simulink library "Lib_EMTAT"  (R2021b)
settings: Solver=VariableStepAuto  StartTime=0.0  StopTime=10.0  RelTol=1e-3
undefined symbols (not defined in the file or in its folder): A_M, B_M, Cj, component_degradation_input, Cs, E0_M, f_sw, K_M, MWS, Q_M, Q_rr, r_c, r_D, R_M, Rj, Ru, SNR_DX_M, SNR_IC_M, SNR_Mn_M, SNR_Mx_M, SOC_Init_M, u_ce0, u_D0
libraries: $bdroot x82, simulink x23, Lib_Dyn_StateSpace_EMTAT x3, PB_Library_Master_Working x1
(part 4 of 7)

== system Lib_EMTAT/Components/Physics-Based/Electrothermal_Battery_Model ==
  note: Electrical Model
  it_base : Inport
  I_Demand : Inport  Port=2
  Temp (Ra) : Inport  Port=3  Unit=degC
  FaultToggle : Inport  Port=4  Unit=degC
  Battery Core (w/ Q) : Subsystem
  Bus Creator : BusCreator  Inputs=7
  Catastrophic Fault Block{,1..5} (6 alike) : $bdroot/Components/Physics-Based/Catastrophic Fault Block  SystemSampleTime=-1  VariantActivationTime=update diagram  Latency=0  AutoFrameSizeCalculation=off
  Degradation Parameter Multiplier : $bdroot/Components/Physics-Based/Degradation Parameter Multiplier  SystemSampleTime=-1  VariantActivationTime=update diagram  Latency=0  AutoFrameSizeCalculation=off
  Product1 : Product
  Rankine to Celsius : $bdroot/Components/Physics-Based/Rankine to Celsius  SystemSampleTime=-1  VariantActivationTime=update diagram  Latency=0  AutoFrameSizeCalculation=off
  it_Dot = f(i) : Subsystem
  Vout : Outport  VectorParamsAs1DForOutWhenUnconnected=off
  Outputs : Outport  Port=2  VectorParamsAs1DForOutWhenUnconnected=off
  it_Dot : Outport  Port=3  VectorParamsAs1DForOutWhenUnconnected=off
  Heat : Outport  Port=4  VectorParamsAs1DForOutWhenUnconnected=off
  SOC : Outport  Port=5  VectorParamsAs1DForOutWhenUnconnected=off
  it : Outport  Port=6  VectorParamsAs1DForOutWhenUnconnected=off
  wires:
  Rankine to Celsius/1 -> Battery Core (w/ Q)/3(Tavg)
  Battery Core (w/ Q)/3(it) -> Catastrophic Fault Block5/2, Bus Creator/6  "it"
  Battery Core (w/ Q)/2(SOC) -> Catastrophic Fault Block4/2, Bus Creator/4  "SOC"
  it_base/1 -> Battery Core (w/ Q)/1(it_base)
  Battery Core (w/ Q)/1(Vout) -> Catastrophic Fault Block/2, Bus Creator/1, Product1/1  "Vout"
  Product1/1 -> Bus Creator/3  "Pout"
  it_Dot = f(i)/1(it_Dot) -> Catastrophic Fault Block2/2, Bus Creator/5  "it_Dot"
  I_Demand/1 -> it_Dot = f(i)/1(i), Battery Core (w/ Q)/2(I_Demand), Bus Creator/2, Product1/2  "Iout"
  Battery Core (w/ Q)/4(Heat_Generated) -> Catastrophic Fault Block3/2, Bus Creator/7  "Heat_Generated"
  Temp (Ra)/1 -> Rankine to Celsius/1
  Catastrophic Fault Block/1 -> Vout/1
  FaultToggle/1 -> [FT]
  [FT] -> Catastrophic Fault Block/1
  [FT] -> Catastrophic Fault Block1/1
  Bus Creator/1 -> Catastrophic Fault Block1/2
  Catastrophic Fault Block1/1 -> Outputs/1
  [FT] -> Catastrophic Fault Block2/1
  Catastrophic Fault Block2/1 -> it_Dot/1
  [FT] -> Catastrophic Fault Block3/1
  Catastrophic Fault Block3/1 -> Heat/1
  Catastrophic Fault Block4/1 -> SOC/1
  [FT] -> Catastrophic Fault Block4/1
  Catastrophic Fault Block5/1 -> it/1
  [FT] -> Catastrophic Fault Block5/1

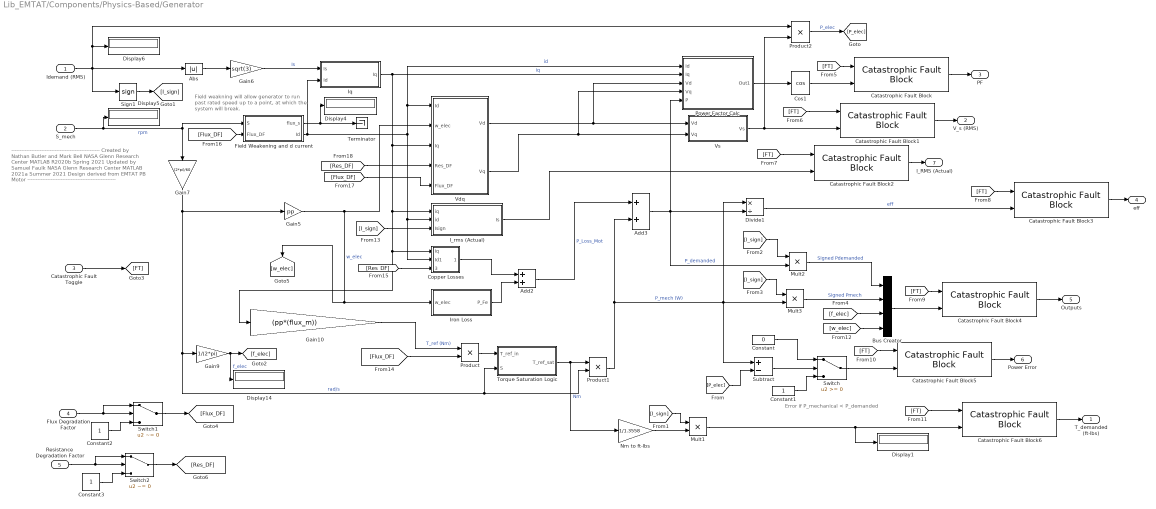
== system Lib_EMTAT/Components/Physics-Based/Generator ==
  note: Field weakning will allow generator to run past rated speed up to a point, at which the system will break.
  note: Error if P_mechanical < P_demanded
  note: -----------------------------------------------------
      | Created by Nathan Butler and Mark Bell
      | NASA Glenn Research Center
      | MATLAB R2020b
      | Spring 2021
      |
      | Updated by Samuel Faulk
      | NASA Glenn Research Center
      | MATLAB 2021a
      | Summer 2021
      |
      | Design derived from EMTAT PB Motor
      | -----------------------------------------------------
  Idemand (RMS) : Inport
  S_mech : Inport  Port=2
  Catastrophic Fault Toggle : Inport  Port=3
  Flux Degradation Factor : Inport  Port=4
  Resistance Degradation Factor : Inport  Port=5
  Abs : Abs
  Add2 : Sum
  Add3 : Sum
  Bus Creator : BusCreator  Inputs=4
  Catastrophic Fault Block{,1..6} (7 alike) : $bdroot/Components/Physics-Based/Catastrophic Fault Block  SystemSampleTime=-1  VariantActivationTime=update diagram  Latency=0  AutoFrameSizeCalculation=off
  Constant : Constant  Value=0
  Constant1 : Constant
  Constant2 : Constant
  Constant3 : Constant
  Copper Losses : Subsystem
  Cos1 : Trigonometry  Operator=cos
  Display{1,4..6,14} (5 alike) : Display
  Divide1 : Product  Inputs=*/
  "Field Weakening and d current " : Subsystem
  Gain10 : Gain  Gain=(pp*(flux_m))
  Gain5 : Gain  Gain=pp
  Gain6 : Gain  Gain=sqrt(3)
  Gain7 : Gain  Gain=(2*pi)/60
  Gain9 : Gain  Gain=1/(2*pi)
  I_rms (Actual) : Subsystem
  Iq : Subsystem
  Iron Loss : Subsystem
  Mult1 : Product  Inputs=**
  Mult2 : Product  Inputs=**
  Mult3 : Product  Inputs=**
  Nm to ft-lbs : Gain  Gain=1/1.3558
  Power Factor Calc : Subsystem
  Product : Product
  Product1 : Product
  Product2 : Product
  Sign1 : Signum
  Subtract : Sum  Inputs=+-
  Switch : Switch
  Switch1 : Switch  Criteria=u2 ~= 0  Threshold=~0
  Switch2 : Switch  Criteria=u2 ~= 0  Threshold=~0
  Terminator : Terminator
  Torque Saturation Logic : Subsystem
  Vdq : Subsystem
  Vs : Subsystem
  T_demanded (ft-lbs) : Outport
  V_s (RMS) : Outport  Port=2
  PF : Outport  Port=3
  eff : Outport  Port=4
  Outputs : Outport  Port=5
  Power Error : Outport  Port=6
  I_RMS (Actual) : Outport  Port=7
  wires:
  Add3/1 -> Power Factor Calc/5(P), Divide1/2, Mult2/2  "P_demanded"
  [w_elec] -> Bus Creator/4
  [f_elec] -> Bus Creator/3
  Gain9/1 -> Display14/1, [f_elec]  "f_elec"
  Mult3/1 -> Bus Creator/2  "Signed Pmech"
  Mult2/1 -> Bus Creator/1  "Signed Pdemanded"
  [I_sign] -> Mult3/1
  [I_sign] -> Mult2/1
  [I_sign] -> Mult1/1
  Sign1/1 -> [I_sign]
  Idemand (RMS)/1 -> Abs/1, Sign1/1, Display6/1, Product2/1
  Torque Saturation Logic/1(T_ref_sat) -> Nm to ft-lbs/1, Product1/1  "Nm"
  Gain6/1 -> Iq/1(Is)  "Is"
  Product1/1 -> Mult3/2, Divide1/1, Subtract/1, Add3/2  "P_mech (W)"
  Iq/1(Iq) -> Power Factor Calc/2(Iq), Gain10/1, Copper Losses/1(Iq), I_rms (Actual)/1(iq), Vdq/3(Iq)  "iq"
  S_mech/1 -> Display5/1, "Field Weakening and d current "/1(S), Gain7/1  "rpm"
  "Field Weakening and d current "/2(Id) -> Copper Losses/2(Id1), I_rms (Actual)/2(id), Power Factor Calc/1(Id), Vdq/1(Id), Iq/2(Id)  "id"
  Gain5/1 -> Iron Loss/1(w_elec), [w_elec], Vdq/2(w_elec)  "w_elec"
  Vdq/1(Vd) -> Vs/1(Vd), Power Factor Calc/3(Vd)
  Vdq/2(Vq) -> Vs/2(Vq), Power Factor Calc/4(Vq)
  Vs/1(Vs) -> Catastrophic Fault Block1/2, Product2/2
  Copper Losses/1(P_Cu) -> Add2/1
  Iron Loss/1(P_Fe) -> Add2/2
  Add2/1 -> Add3/1  "P_Loss_Mot"
  Power Factor Calc/1(Out1) -> Cos1/1
  Subtract/1 -> Switch/2
  Constant/1 -> Switch/1
  Constant1/1 -> Switch/3
  Product2/1 -> [P_elec]  "P_elec"
  [P_elec] -> Subtract/2
  Nm to ft-lbs/1 -> Mult1/2
  Gain7/1 -> Gain5/1, Gain9/1, Torque Saturation Logic/2(S), Product1/2  "rad/s"
  Abs/1 -> Gain6/1
  [FT] -> Catastrophic Fault Block/1
  Cos1/1 -> Catastrophic Fault Block/2
  Catastrophic Fault Block/1 -> PF/1
  [FT] -> Catastrophic Fault Block1/1
  Catastrophic Fault Block1/1 -> V_s (RMS)/1
  [FT] -> Catastrophic Fault Block2/1
  Catastrophic Fault Block2/1 -> I_RMS (Actual)/1
  I_rms (Actual)/1(Is) -> Catastrophic Fault Block2/2
  [FT] -> Catastrophic Fault Block3/1
  Divide1/1 -> Catastrophic Fault Block3/2  "eff"
  Catastrophic Fault Block3/1 -> eff/1
  [FT] -> Catastrophic Fault Block4/1
  Bus Creator/1 -> Catastrophic Fault Block4/2
  Catastrophic Fault Block4/1 -> Outputs/1
  [FT] -> Catastrophic Fault Block5/1
  Switch/1 -> Catastrophic Fault Block5/2
  Catastrophic Fault Block5/1 -> Power Error/1
  [FT] -> Catastrophic Fault Block6/1
  Mult1/1 -> Display1/1, Catastrophic Fault Block6/2
  Catastrophic Fault Block6/1 -> T_demanded (ft-lbs)/1
  [I_sign] -> I_rms (Actual)/3(Isign)
  Catastrophic Fault Toggle/1 -> [FT]
  Product/1 -> Torque Saturation Logic/1(T_ref_in)
  Gain10/1 -> Product/1  "T_ref (Nm)"
  Constant2/1 -> Switch1/3
  Flux Degradation Factor/1 -> Switch1/2, Switch1/1
  Switch1/1 -> [Flux_DF]
  [Flux_DF] -> Product/2
  Resistance Degradation Factor/1 -> Switch2/2, Switch2/1
  Constant3/1 -> Switch2/3
  Switch2/1 -> [Res_DF]
  "Field Weakening and d current "/1(flux_s) -> Terminator/1, Display4/1
  [Flux_DF] -> "Field Weakening and d current "/2(Flux_DF)
  [Res_DF] -> Copper Losses/3(Res_DF)
  [Res_DF] -> Vdq/4(Res_DF)
  [Flux_DF] -> Vdq/5(Flux_DF)

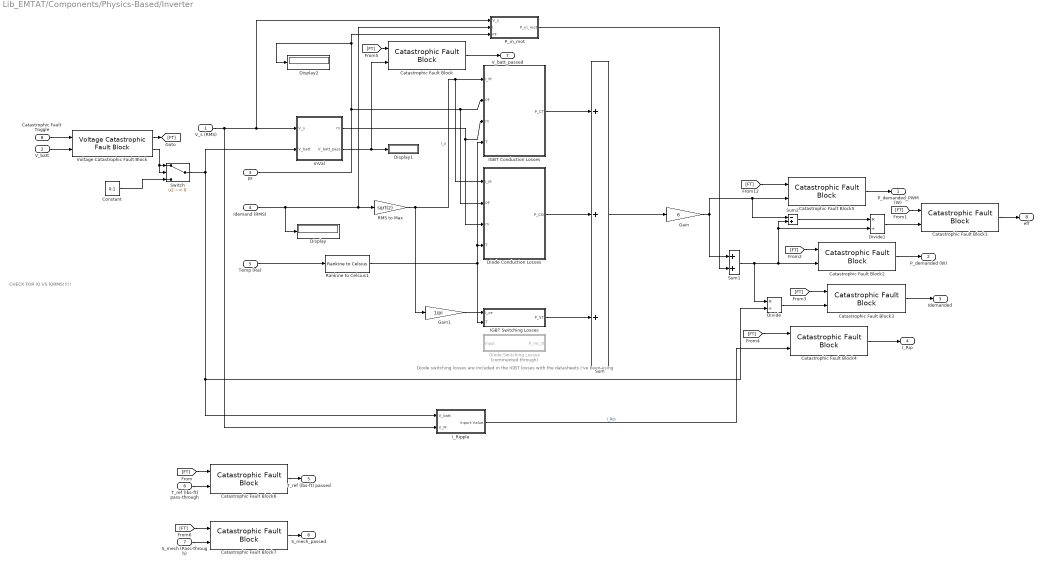
== system Lib_EMTAT/Components/Physics-Based/Inverter  ==
  note: Diode switching losses are included in the IGBT losses with the datasheets I've been using
  note: CHECK FOR IO VS IORMS!!!!!
  "V_s (RMS) " : Inport
  V_batt : Inport  Port=2
  PF : Inport  Port=3
  Idemand (RMS) : Inport  Port=4
  Temp (Ra) : Inport  Port=5
  T_ref (lbs-ft) pass-through : Inport  Port=6
  S_mech (Pass-through) : Inport  Port=7
  Catastrophic Fault Toggle : Inport  Port=8
  Catastrophic Fault Block{,1..7} (8 alike) : $bdroot/Components/Physics-Based/Catastrophic Fault Block  SystemSampleTime=-1  VariantActivationTime=update diagram  Latency=0  AutoFrameSizeCalculation=off
  Constant : Constant  Value=0.1
  Diode Conduction Losses : Subsystem
  Diode Switching Losses : Subsystem  Commented=through
  Display : Display
  Display1 : Display
  Display2 : Display
  Divide : Product  Inputs=*/
  Divide1 : Product  Inputs=*/
  Gain : Gain  Gain=6
  Gain1 : Gain  Gain=1/pi
  IGBT Conduction Losses : Subsystem
  IGBT Switching Losses : Subsystem
  I_Ripple : Subsystem
  P_in_mot : Subsystem
  RMS to Max : Gain  Gain=sqrt(2)
  Rankine to Celsius1 : $bdroot/Components/Physics-Based/Rankine to Celsius  SystemSampleTime=-1  VariantActivationTime=update diagram  Latency=0  AutoFrameSizeCalculation=off
  Sum : Sum  Inputs=+++
  Sum1 : Sum
  Sum2 : Sum  Inputs=-+
  Switch : Switch  Criteria=u2 ~= 0
  Voltage Catastrophic Fault Block : $bdroot/Components/Physics-Based/Voltage Catastrophic Fault Block  SystemSampleTime=-1  VariantActivationTime=update diagram  Latency=0  AutoFrameSizeCalculation=off
  mVal : Subsystem
  P_demanded_PWM (W) : Outport  VectorParamsAs1DForOutWhenUnconnected=off
  P_demanded (W) : Outport  Port=2  VectorParamsAs1DForOutWhenUnconnected=off
  Idemanded : Outport  Port=3  VectorParamsAs1DForOutWhenUnconnected=off
  I_Rip : Outport  Port=4  VectorParamsAs1DForOutWhenUnconnected=off
  T_ref (lbs-ft) passed : Outport  Port=5  VectorParamsAs1DForOutWhenUnconnected=off
  S_mech_passed : Outport  Port=6  VectorParamsAs1DForOutWhenUnconnected=off
  V_batt_passed : Outport  Port=7  VectorParamsAs1DForOutWhenUnconnected=off
  eff : Outport  Port=8  VectorParamsAs1DForOutWhenUnconnected=off
  wires:
  RMS to Max/1 -> Gain1/1, Diode Conduction Losses/1(I_M), IGBT Conduction Losses/1(I_M)  "I_o"
  IGBT Conduction Losses/1(P_CT) -> Sum/1
  Sum/1 -> Gain/1
  Gain/1 -> Sum1/1, Catastrophic Fault Block5/2, Sum2/1
  PF/1 -> P_in_mot/3(PF), Display2/1, Diode Conduction Losses/2(PF), IGBT Conduction Losses/2(PF)
  mVal/1(m) -> Diode Conduction Losses/3(m), IGBT Conduction Losses/3(m)
  P_in_mot/1(P_in_mot) -> Sum1/2
  Gain1/1 -> IGBT Switching Losses/1(I_ce)
  IGBT Switching Losses/1(P_ST) -> Sum/3
  Diode Conduction Losses/1(P_CD) -> Sum/2
  Temp (Ra)/1 -> Rankine to Celsius1/1
  Sum1/1 -> Divide/1, Catastrophic Fault Block2/2, Sum2/2, Divide1/2
  Sum2/1 -> Divide1/1
  Rankine to Celsius1/1 -> IGBT Switching Losses/2(T), Diode Conduction Losses/4(T), IGBT Conduction Losses/4(T)
  [FT] -> Catastrophic Fault Block5/1
  Catastrophic Fault Block5/1 -> P_demanded_PWM (W)/1
  [FT] -> Catastrophic Fault Block1/1
  Divide1/1 -> Catastrophic Fault Block1/2
  Catastrophic Fault Block1/1 -> eff/1
  [FT] -> Catastrophic Fault Block2/1
  Catastrophic Fault Block2/1 -> P_demanded (W)/1
  [FT] -> Catastrophic Fault Block3/1
  Divide/1 -> Catastrophic Fault Block3/2
  Catastrophic Fault Block3/1 -> Idemanded/1
  [FT] -> Catastrophic Fault Block4/1
  I_Ripple/1(Inport Value) -> Catastrophic Fault Block4/2  "I_Rip"
  Catastrophic Fault Block4/1 -> I_Rip/1
  "V_s (RMS) "/1 -> mVal/1(V_s), P_in_mot/1(V_s), I_Ripple/2("V_M ")
  Catastrophic Fault Block/1 -> V_batt_passed/1
  [FT] -> Catastrophic Fault Block/1
  mVal/2(V_batt_pass) -> Catastrophic Fault Block/2, Display1/1
  Switch/1 -> mVal/2(V_batt), I_Ripple/1(V_batt), Divide/2
  V_batt/1 -> Voltage Catastrophic Fault Block/2
  Catastrophic Fault Toggle/1 -> Voltage Catastrophic Fault Block/1
  Voltage Catastrophic Fault Block/1 -> [FT]
  T_ref (lbs-ft) pass-through/1 -> Catastrophic Fault Block6/2
  Catastrophic Fault Block6/1 -> T_ref (lbs-ft) passed/1
  [FT] -> Catastrophic Fault Block6/1
  [FT] -> Catastrophic Fault Block7/1
  S_mech (Pass-through)/1 -> Catastrophic Fault Block7/2
  Catastrophic Fault Block7/1 -> S_mech_passed/1
  Idemand (RMS)/1 -> RMS to Max/1, P_in_mot/2(I), Display/1
  Constant/1 -> Switch/3
  Voltage Catastrophic Fault Block/2 -> Switch/1, Switch/2

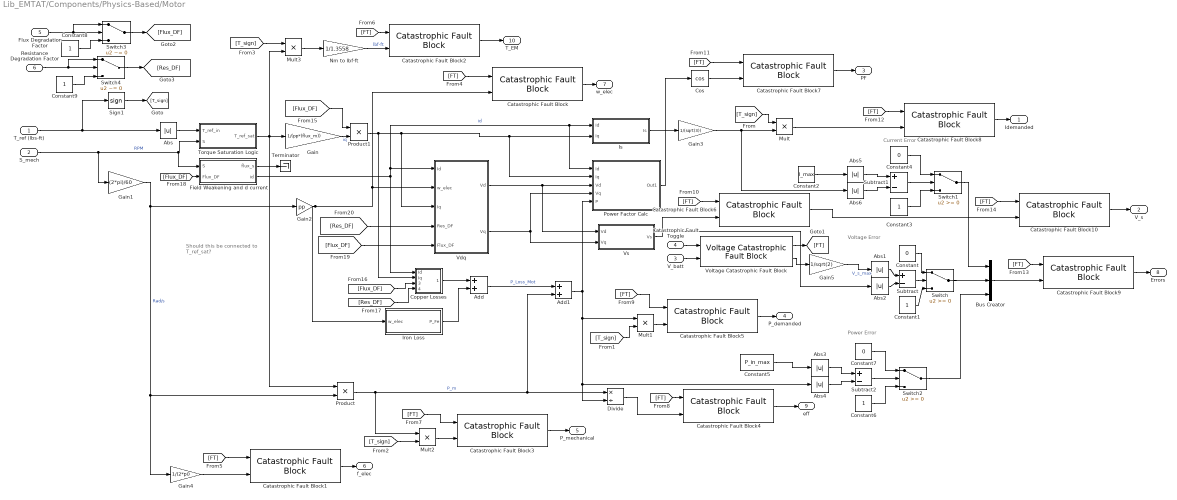
== system Lib_EMTAT/Components/Physics-Based/Motor  ==
  note: Voltage Error
  note: Current Error
  note: Should this be connected
      | to T_ref_sat?
  note: Power Error
  T_ref (lbs-ft) : Inport
  S_mech : Inport  Port=2
  V_batt : Inport  Port=3
  Catastrophic Fault Toggle : Inport  Port=4
  Flux Degradation Factor : Inport  Port=5
  Resistance Degradation Factor : Inport  Port=6
  Abs{,1..6} (7 alike) : Abs
  Add : Sum
  Add1 : Sum
  Bus Creator : BusCreator  Inputs=3
  Catastrophic Fault Block{,1..10} (11 alike) : $bdroot/Components/Physics-Based/Catastrophic Fault Block  SystemSampleTime=-1  VariantActivationTime=update diagram  Latency=0  AutoFrameSizeCalculation=off
  Constant : Constant  Value=0
  Constant{1,3,6,8..9} (5 alike) : Constant
  Constant2 : Constant  Value=I_max
  Constant4 : Constant  Value=0
  Constant5 : Constant  Value=P_in_max
  Constant7 : Constant  Value=0
  Copper Losses : Subsystem
  Cos : Trigonometry  Operator=cos
  Divide : Product  Inputs=*/
  "Field Weakening and d current " : Subsystem
  Gain : Gain  Gain=1/(pp*(flux_m))
  Gain1 : Gain  Gain=(2*pi)/60
  Gain2 : Gain  Gain=pp
  Gain3 : Gain  Gain=1/(sqrt(3))
  Gain4 : Gain  Gain=1/(2*pi)
  Gain5 : Gain  Gain=1/sqrt(2)
  Iron Loss : Subsystem
  Is : Subsystem
  Mult{,1..3} (4 alike) : Product  Inputs=**
  Nm to lbf-ft : Gain  Gain=1/1.3558
  "Power Factor Calc " : Subsystem
  Product : Product
  Product1 : Product
  Sign1 : Signum
  Subtract : Sum  Inputs=+-
  Subtract1 : Sum  Inputs=+-
  Subtract2 : Sum  Inputs=+-
  Switch : Switch
  Switch1 : Switch
  Switch2 : Switch
  Switch3 : Switch  Criteria=u2 ~= 0  Threshold=~0
  Switch4 : Switch  Criteria=u2 ~= 0  Threshold=~0
  Terminator : Terminator
  Torque Saturation Logic : Subsystem
  Vdq : Subsystem
  Voltage Catastrophic Fault Block : $bdroot/Components/Physics-Based/Voltage Catastrophic Fault Block  SystemSampleTime=-1  VariantActivationTime=update diagram  Latency=0  AutoFrameSizeCalculation=off
  Vs : Subsystem
  Idemanded : Outport  VectorParamsAs1DForOutWhenUnconnected=off
  V_s : Outport  Port=2  VectorParamsAs1DForOutWhenUnconnected=off
  PF : Outport  Port=3  VectorParamsAs1DForOutWhenUnconnected=off
  P_demanded : Outport  Port=4  VectorParamsAs1DForOutWhenUnconnected=off
  P_mechanical : Outport  Port=5  VectorParamsAs1DForOutWhenUnconnected=off
  f_elec : Outport  Port=6  VectorParamsAs1DForOutWhenUnconnected=off
  w_elec : Outport  Port=7  VectorParamsAs1DForOutWhenUnconnected=off
  Errors : Outport  Port=8  VectorParamsAs1DForOutWhenUnconnected=off
  eff : Outport  Port=9  VectorParamsAs1DForOutWhenUnconnected=off
  T_EM : Outport  Port=10  VectorParamsAs1DForOutWhenUnconnected=off
  wires:
  [T_sign] -> Mult3/1
  [T_sign] -> Mult2/2
  [T_sign] -> Mult1/2
  Abs/1 -> Torque Saturation Logic/1(T_ref_in)
  Add/1 -> Add1/1  "P_Loss_Mot"
  Add1/1 -> Abs4/1, Divide/2, Mult1/1, "Power Factor Calc "/5(P)
  [T_sign] -> Mult/1
  Sign1/1 -> [T_sign]
  "Field Weakening and d current "/2(id) -> "Power Factor Calc "/1(Id), Is/1(Id), Vdq/1(Id), Copper Losses/1(Id)  "id"
  Gain3/1 -> Abs6/1, Mult/2
  Gain2/1 -> Catastrophic Fault Block/2, Vdq/2(w_elec), Iron Loss/1(w_elec)
  Torque Saturation Logic/1(T_ref_sat) -> Gain/1, Product/1, Mult3/2
  Gain1/1 -> Product/2, Gain4/1, Gain2/1  "Rad/s"
  Copper Losses/1(P_Cu) -> Add/1
  Iron Loss/1(P_Fe) -> Add/2
  Product/1 -> Divide/1, Add1/2, Mult2/1  "P_m"
  Vdq/1(Vd) -> "Power Factor Calc "/3(Vd), Vs/1(Vd)
  Vdq/2(Vq) -> "Power Factor Calc "/4(Vq), Vs/2(Vq)
  Is/1(Is) -> Gain3/1
  Vs/1(Vs) -> Catastrophic Fault Block6/2, Abs2/1
  "Power Factor Calc "/1(Out1) -> Cos/1
  Gain5/1 -> Abs1/1  "V_s_max"
  Subtract/1 -> Switch/2
  Constant/1 -> Switch/1
  Constant1/1 -> Switch/3
  Switch/1 -> Bus Creator/2
  Constant2/1 -> Abs5/1
  Switch1/1 -> Bus Creator/1
  Constant3/1 -> Switch1/3
  Constant4/1 -> Switch1/1
  Subtract1/1 -> Switch1/2
  Constant7/1 -> Switch2/1
  Constant5/1 -> Abs3/1
  Subtract2/1 -> Switch2/2
  Constant6/1 -> Switch2/3
  Switch2/1 -> Bus Creator/3
  Catastrophic Fault Block/1 -> w_elec/1
  [FT] -> Catastrophic Fault Block/1
  [FT] -> Catastrophic Fault Block1/1
  Gain4/1 -> Catastrophic Fault Block1/2
  Catastrophic Fault Block1/1 -> f_elec/1
  [FT] -> Catastrophic Fault Block2/1
  Mult3/1 -> Nm to lbf-ft/1
  Catastrophic Fault Block2/1 -> T_EM/1
  [FT] -> Catastrophic Fault Block3/1
  Mult2/1 -> Catastrophic Fault Block3/2
  Catastrophic Fault Block3/1 -> P_mechanical/1
  [FT] -> Catastrophic Fault Block4/1
  Divide/1 -> Catastrophic Fault Block4/2
  Catastrophic Fault Block4/1 -> eff/1
  [FT] -> Catastrophic Fault Block5/1
  Mult1/1 -> Catastrophic Fault Block5/2
  Catastrophic Fault Block5/1 -> P_demanded/1
  [FT] -> Catastrophic Fault Block6/1
  [FT] -> Catastrophic Fault Block7/1
  Cos/1 -> Catastrophic Fault Block7/2
  Catastrophic Fault Block7/1 -> PF/1
  [FT] -> Catastrophic Fault Block8/1
  Mult/1 -> Catastrophic Fault Block8/2
  Catastrophic Fault Block8/1 -> Idemanded/1
  [FT] -> Catastrophic Fault Block9/1
  Bus Creator/1 -> Catastrophic Fault Block9/2
  Catastrophic Fault Block9/1 -> Errors/1
  [FT] -> Catastrophic Fault Block10/1
  Catastrophic Fault Block6/1 -> Catastrophic Fault Block10/2
  Catastrophic Fault Block10/1 -> V_s/1
  "Field Weakening and d current "/1(flux_s) -> Terminator/1
  Gain/1 -> Product1/2  "iq"
  Product1/1 -> Copper Losses/2(Iq), Vdq/3(Iq), "Power Factor Calc "/2(Iq), Is/2(Iq)
  T_ref (lbs-ft)/1 -> Sign1/1, Abs/1
  S_mech/1 -> Gain1/1, "Field Weakening and d current "/1(S), Torque Saturation Logic/2(S)  "RPM"
  Voltage Catastrophic Fault Block/2 -> Gain5/1
  Catastrophic Fault Toggle/1 -> Voltage Catastrophic Fault Block/1
  Voltage Catastrophic Fault Block/1 -> [FT]
  V_batt/1 -> Voltage Catastrophic Fault Block/2
  Constant8/1 -> Switch3/3
  Flux Degradation Factor/1 -> Switch3/2, Switch3/1
  Switch3/1 -> [Flux_DF]
  [Flux_DF] -> Product1/1
  Resistance Degradation Factor/1 -> Switch4/2, Switch4/1
  Constant9/1 -> Switch4/3
  Switch4/1 -> [Res_DF]
  [Flux_DF] -> Copper Losses/3(Flux_DF)
  [Res_DF] -> Copper Losses/4(Res_DF)
  [Flux_DF] -> "Field Weakening and d current "/2(Flux_DF)
  [Res_DF] -> Vdq/4(Res_DF)
  [Flux_DF] -> Vdq/5(Flux_DF)
  Abs1/1 -> Subtract/1
  Abs2/1 -> Subtract/2
  Abs3/1 -> Subtract2/1
  Abs4/1 -> Subtract2/2
  Abs5/1 -> Subtract1/1
  Abs6/1 -> Subtract1/2
  Nm to lbf-ft/1 -> Catastrophic Fault Block2/2  "lbf-ft"

== system Lib_EMTAT/Components/Physics-Based/Rankine to Celsius ==
  Rankine : Inport
  Add : Sum  Inputs=+-
  Constant : Constant  Value=491.67
  Constant1 : Constant  Value=1.8
  Divide : Product  Inputs=*/
  Celsius : Outport
  wires:
  Constant1/1 -> Divide/2
  Add/1 -> Divide/1
  Constant/1 -> Add/2
  Rankine/1 -> Add/1
  Divide/1 -> Celsius/1

== system Lib_EMTAT/Components/Physics-Based/Rectifier ==
  note: -------------------------------------------------------
      | Created by Nathan Butler and Mark Bell
      | NASA Glenn Research Center
      | MATLAB R2020b
      | Spring 2021
      |
      | Design derived from EMTAT PB Inverter
      | -------------------------------------------------------
  Idemand : Inport
  "V_s (RMS) " : Inport  Port=2
  PF : Inport  Port=3
  Temp (Ra) : Inport  Port=4
  V_batt (Standin) : Inport  Port=5
  Catastrophic Fault Toggle : Inport  Port=6
  Catastrophic Fault Block{,1..5} (6 alike) : $bdroot/Components/Physics-Based/Catastrophic Fault Block  SystemSampleTime=-1  VariantActivationTime=update diagram  Latency=0  AutoFrameSizeCalculation=off
  Constant : Constant  Value=0.1
  Diode Conduction Losses1 : Subsystem
  Display : Display
  Divide2 : Product  Inputs=*/
  Divide3 : Product  Inputs=*/
  Gain2 : Gain  Gain=6
  Gain3 : Gain  Gain=1/pi
  IGBT Conduction Losses1 : Subsystem
  IGBT Switching Losses1 : Subsystem
  I_Ripple1 : Subsystem
  Math : Gain  Gain=1/sqrt(2)
  P_out_gen : Subsystem
  "RMS to V_batt " : Gain  Gain=sqrt(2)
  Rankine to Celsius : $bdroot/Components/Physics-Based/Rankine to Celsius  SystemSampleTime=-1  VariantActivationTime=update diagram  Latency=0  AutoFrameSizeCalculation=off
  Sum3 : Sum
  Sum4 : Sum  Inputs=+++
  Sum5 : Sum  Inputs=-+
  Switch : Switch  Criteria=u2 ~= 0
  Terminator : Terminator
  Voltage Catastrophic Fault Block : $bdroot/Components/Physics-Based/Voltage Catastrophic Fault Block  SystemSampleTime=-1  VariantActivationTime=update diagram  Latency=0  AutoFrameSizeCalculation=off
  mVal : Subsystem
  to I_RMS : Gain  Commented=through  Gain=1/sqrt(2)
  P_demanded_PWM (W) : Outport  VectorParamsAs1DForOutWhenUnconnected=off
  P_demanded (W) : Outport  Port=2  VectorParamsAs1DForOutWhenUnconnected=off
  Idemanded (RMS) : Outport  Port=3  VectorParamsAs1DForOutWhenUnconnected=off
  I_Rip : Outport  Port=4  VectorParamsAs1DForOutWhenUnconnected=off
  V_out : Outport  Port=5  VectorParamsAs1DForOutWhenUnconnected=off
  eff : Outport  Port=6  VectorParamsAs1DForOutWhenUnconnected=off
  wires:
  Math/1 -> Divide2/1
  [V_S_RMS] -> Divide2/2
  Switch/1 -> "RMS to V_batt "/1, I_Ripple1/2("V_M "), mVal/1(V_s), [V_S_RMS]
  Rankine to Celsius/1 -> IGBT Conduction Losses1/4(T), IGBT Switching Losses1/2(T), Diode Conduction Losses1/4(T)
  "RMS to V_batt "/1 -> Catastrophic Fault Block4/2, I_Ripple1/1(V_batt), mVal/2(V_batt), P_out_gen/2(V_s (DC))  "V_batt"
  Divide2/1 -> Catastrophic Fault Block3/2  "Idemanded"
  P_out_gen/1(P_out_gen) -> Sum3/1, Display/1  "P_out_gen"
  Gain2/1 -> Sum3/2, Catastrophic Fault Block/2, Sum5/1  "P_demanded_PWM"
  Idemand/1 -> IGBT Conduction Losses1/1(I_M), Gain3/1, Diode Conduction Losses1/1(I_M), to I_RMS/1  "Idemand"
  PF/1 -> P_out_gen/3(PF), Diode Conduction Losses1/2(PF), IGBT Conduction Losses1/2(PF)  "PF"
  mVal/1(m) -> Diode Conduction Losses1/3(m), IGBT Conduction Losses1/3(m)  "(=1)"
  Diode Conduction Losses1/1(P_CD) -> Sum4/2
  Sum4/1 -> Gain2/1
  IGBT Conduction Losses1/1(P_CT) -> Sum4/1
  IGBT Switching Losses1/1(P_ST) -> Sum4/3
  Gain3/1 -> IGBT Switching Losses1/1(I_ce)
  Temp (Ra)/1 -> Rankine to Celsius/1  "Temp (Ra)"
  Sum3/1 -> Catastrophic Fault Block2/2, Divide3/2, Sum5/2, Math/1  "P_demanded"
  Sum5/1 -> Divide3/1
  to I_RMS/1 -> P_out_gen/1(I (DC))
  V_batt (Standin)/1 -> Terminator/1  "V_batt"
  Catastrophic Fault Block/1 -> P_demanded_PWM (W)/1
  [FT] -> Catastrophic Fault Block/1
  [FT] -> Catastrophic Fault Block1/1
  Divide3/1 -> Catastrophic Fault Block1/2  "eff"
  Catastrophic Fault Block1/1 -> eff/1
  [FT] -> Catastrophic Fault Block2/1
  Catastrophic Fault Block2/1 -> P_demanded (W)/1
  [FT] -> Catastrophic Fault Block3/1
  Catastrophic Fault Block3/1 -> Idemanded (RMS)/1
  [FT] -> Catastrophic Fault Block4/1
  Catastrophic Fault Block4/1 -> V_out/1
  [FT] -> Catastrophic Fault Block5/1
  I_Ripple1/1(I_Rip) -> Catastrophic Fault Block5/2  "I_Rip"
  Catastrophic Fault Block5/1 -> I_Rip/1
  Voltage Catastrophic Fault Block/1 -> [FT]
  Catastrophic Fault Toggle/1 -> Voltage Catastrophic Fault Block/1
  "V_s (RMS) "/1 -> Voltage Catastrophic Fault Block/2  "V_s (RMS)"
  Constant/1 -> Switch/3
  Voltage Catastrophic Fault Block/2 -> Switch/1, Switch/2

== system Lib_EMTAT/Components/Physics-Based/Resistor Current Control ==
  Idemand : Inport
  Resistance : Inport  Port=2
  Temp (Rankine) : Inport  Port=3  Unit=degC
  FaultToggle : Inport  Port=4  Unit=degC
  Degredation : Inport  Port=5
  Catastrophic Fault Block : $bdroot/Components/Physics-Based/Catastrophic Fault Block  SystemSampleTime=-1  VariantActivationTime=update diagram  Latency=0  AutoFrameSizeCalculation=off
  Catastrophic Fault Block1 : $bdroot/Components/Physics-Based/Catastrophic Fault Block  SystemSampleTime=-1  VariantActivationTime=update diagram  Latency=0  AutoFrameSizeCalculation=off
  Catastrophic Fault Block2 : $bdroot/Components/Physics-Based/Catastrophic Fault Block  SystemSampleTime=-1  VariantActivationTime=update diagram  Latency=0  AutoFrameSizeCalculation=off
  Constant : Constant
  Multiply : Product
  Multiply1 : Product
  Product1 : Product
  Rankine to Celsius : $bdroot/Components/Physics-Based/Rankine to Celsius  SystemSampleTime=-1  VariantActivationTime=update diagram  Latency=0  AutoFrameSizeCalculation=off
  Switch : Switch  Criteria=u2 ~= 0  Threshold=~0
  Terminator : Terminator
  VDrop : Outport  VectorParamsAs1DForOutWhenUnconnected=off
  Idemanded : Outport  Port=2  VectorParamsAs1DForOutWhenUnconnected=off
  Heat : Outport  Port=3  VectorParamsAs1DForOutWhenUnconnected=off
  wires:
  Multiply/1 -> Catastrophic Fault Block/2, Multiply1/1
  Temp (Rankine)/1 -> Rankine to Celsius/1
  Rankine to Celsius/1 -> Terminator/1
  FaultToggle/1 -> [FT]
  [FT] -> Catastrophic Fault Block/1
  Catastrophic Fault Block/1 -> VDrop/1
  [FT] -> Catastrophic Fault Block1/1
  Catastrophic Fault Block1/1 -> Idemanded/1
  [FT] -> Catastrophic Fault Block2/1
  Multiply1/1 -> Catastrophic Fault Block2/2
  Catastrophic Fault Block2/1 -> Heat/1
  Idemand/1 -> Catastrophic Fault Block1/2, Multiply1/2, Multiply/2
  Degredation/1 -> Switch/2, Switch/1
  Resistance/1 -> Product1/2
  Product1/1 -> Multiply/1
  Constant/1 -> Switch/3
  Switch/1 -> Product1/1

== system Lib_EMTAT/Components/Physics-Based/Resistor Voltage Control ==
  "VDrop " : Inport
  "Resistance " : Inport  Port=2
  Temp : Inport  Port=3  Unit=degC
  FaultToggle : Inport  Port=4  Unit=degC
  Degredation : Inport  Port=5
  Catastrophic Fault Block : $bdroot/Components/Physics-Based/Catastrophic Fault Block  SystemSampleTime=-1  VariantActivationTime=update diagram  Latency=0  AutoFrameSizeCalculation=off
  Catastrophic Fault Block1 : $bdroot/Components/Physics-Based/Catastrophic Fault Block  SystemSampleTime=-1  VariantActivationTime=update diagram  Latency=0  AutoFrameSizeCalculation=off
  Constant : Constant
  Divide : Product  Inputs=*/
  Multiply1 : Product
  Product : Product
  Rankine to Celsius : $bdroot/Components/Physics-Based/Rankine to Celsius  SystemSampleTime=-1  VariantActivationTime=update diagram  Latency=0  AutoFrameSizeCalculation=off
  Switch : Switch  Criteria=u2 ~= 0  Threshold=~0
  Terminator : Terminator
  Idemand : Outport  VectorParamsAs1DForOutWhenUnconnected=off
  Heat : Outport  Port=2  VectorParamsAs1DForOutWhenUnconnected=off
  wires:
  "VDrop "/1 -> Multiply1/1, Divide/1
  Divide/1 -> Catastrophic Fault Block/2, Multiply1/2
  Temp/1 -> Rankine to Celsius/1
  Rankine to Celsius/1 -> Terminator/1
  FaultToggle/1 -> [FT]
  [FT] -> Catastrophic Fault Block/1
  Catastrophic Fault Block/1 -> Idemand/1
  Multiply1/1 -> Catastrophic Fault Block1/2
  [FT] -> Catastrophic Fault Block1/1
  Catastrophic Fault Block1/1 -> Heat/1
  Product/1 -> Divide/2
  "Resistance "/1 -> Product/2
  Switch/1 -> Product/1
  Constant/1 -> Switch/3
  Degredation/1 -> Switch/2, Switch/1

== system Lib_EMTAT/Components/Physics-Based/Temperature Calculation Block ==
  Heat_Generated : Inport
  T_ambient : Inport  Port=2  Unit=degR
  1/Cj_M : Gain  Gain=1/Cj_M
  1/Cs_M : Gain  Gain=1/Cs_M
  1/Rj_M : Gain  Gain=1/Rj_M
  1/Ru_M : Gain  Gain=1/Ru_M
  Sum : Sum  Inputs=|-+
  Sum1 : Sum  Inputs=|++
  Sum2 : Sum  Inputs=|-+
  Sum3 : Sum  Inputs=|-+
  Tj : Integrator  InitialCondition=Tj_0_M
  Ts : Integrator  InitialCondition=Ts_0_M
  T_Junction : Outport  VectorParamsAs1DForOutWhenUnconnected=off
  T_surface : Outport  Port=2  VectorParamsAs1DForOutWhenUnconnected=off
  wires:
  Ts/1 -> Sum3/1, T_surface/1, Sum/2  "T_Surface"
  Tj/1 -> Sum/1, T_Junction/1  "T_Junction"
  T_ambient/1 -> Sum3/2
  Heat_Generated/1 -> Sum1/1
  Sum/1 -> 1/Rj_M/1
  1/Rj_M/1 -> Sum2/1, Sum1/2
  Sum1/1 -> 1/Cj_M/1
  1/Cj_M/1 -> Tj/1
  Sum2/1 -> 1/Cs_M/1
  1/Cs_M/1 -> Ts/1
  Sum3/1 -> 1/Ru_M/1
  1/Ru_M/1 -> Sum2/2

== system Lib_EMTAT/Components/Physics-Based/Voltage Catastrophic Fault Block ==
  Inport Fault Toggle : Inport
  Inport Voltage : Inport  Port=2
  Display{,1..3} (4 alike) : Display
  IsNonZero : simulink/Logic and Bit Operations/Compare To Zero  relop=~=  OutDataTypeStr=boolean
  IsZero : simulink/Logic and Bit Operations/Compare To Zero  relop===  OutDataTypeStr=boolean
  IsZero1 : simulink/Logic and Bit Operations/Compare To Zero  relop===  OutDataTypeStr=boolean
  OR : Logic  Operator=OR  IconShape=distinctive  AllPortsSameDT=off  OutDataTypeStr=boolean
  Switch : Switch  Criteria=u2 > Threshold
  Switch1 : Switch  Criteria=u2 > Threshold
  Zero1 : Constant
  Zero2 : Constant  Value=0
  Outport Fault Toggle : Outport
  Outport Voltage : Outport  Port=2
  wires:
  Switch1/1 -> Outport Voltage/1, Display3/1, IsZero1/1
  Inport Voltage/1 -> IsZero/1, Switch1/3
  Zero2/1 -> Switch1/1
  IsZero1/1 -> Switch/2
  Switch/1 -> Outport Fault Toggle/1, Display1/1
  [FT] -> Switch/3
  Zero1/1 -> Switch/1
  IsZero/1 -> Display2/1, OR/2
  IsNonZero/1 -> OR/1, Display/1
  OR/1 -> Switch1/2
  Inport Fault Toggle/1 -> [FT]
  [FT] -> IsNonZero/1

== system Lib_EMTAT/Components/Power Flow/AC-AC Transformer ==
  V_LN_rms_1 : Inport
  I_L_rms_2 : Inport  Port=2
  Fail? : Inport  Port=3
  Deg : Inport  Port=4
  Bus Creator1 : BusCreator  Inputs=8
  Compensate for Divide By Zero : Subsystem
  Direction Determination : Subsystem
  Divide1 : Product  Inputs=**
  Divide3 : Product  Inputs=**
  Efficiency : Subsystem
  Failure Determination : Subsystem
  Open Circuit Failure - DC Current : Subsystem
  Open Circuit Failure - Line to Neutral Voltage : Subsystem
  Open Circuit/ Degradation Failure : Subsystem
  Power Loss : Subsystem
  Transformer Ratio : Gain  Gain=K
  V_LN_rms_2 : Outport
  Outputs : Outport  Port=2
  Ploss : Outport  Port=3
  I_L_rms_1 : Outport  Port=4
  wires:
  Compensate for Divide By Zero/1(I_L_rms_1) -> Open Circuit Failure - DC Current/2(I_L_rms_1)
  V_LN_rms_1/1 -> [V_LN_rms_1], Power Loss/1(V_LN_rms_1), Compensate for Divide By Zero/2(V_LN_rms_1), Divide1/2, Transformer Ratio/1
  Divide1/1 -> [P_AC_1]
  Direction Determination/1(P_AC_1) -> Compensate for Divide By Zero/1(P_AC_1)
  Bus Creator1/1 -> Outputs/1
  [P_AC_2] -> Bus Creator1/1  "P_AC_2"
  [P_AC_1] -> Bus Creator1/2  "P_AC_1"
  Open Circuit/ Degradation Failure/1("Ploss ") -> Direction Determination/2(Ploss), [Ploss]
  Open Circuit Failure - DC Current/1("I_L_rms_1 ") -> Divide1/1, I_L_rms_1/1, [I_L_rms_1]
  Divide3/1 -> Direction Determination/1(P_AC_2), [P_AC_2]
  [Ploss] -> Ploss/1
  I_L_rms_2/1 -> Power Loss/2(I_L_rms_2), Divide3/2, [I_L_rms_2]
  [V_LN_rms_2] -> Bus Creator1/4  "V_LN_rms_2"
  [V_LN_rms_1] -> Bus Creator1/5  "V_LN_rms_1"
  [I_L_rms_1] -> Bus Creator1/7  "I_L_rms_1"
  [Ploss] -> Bus Creator1/8  "Ploss"
  [I_L_rms_2] -> Bus Creator1/6  "I_L_rms_2"
  [P_AC_1] -> Efficiency/2(P_AC_1)
  [P_AC_2] -> Efficiency/1(P_AC_2)
  Efficiency/1(Eff) -> [Eff]
  [Eff] -> Bus Creator1/3  "Eff"
  [OCFail] -> Open Circuit Failure - DC Current/1(Failed?)
  Transformer Ratio/1 -> Open Circuit Failure - Line to Neutral Voltage/2(V_LN_rms_2)
  [OCFail] -> Open Circuit Failure - Line to Neutral Voltage/1(Failed?)
  Open Circuit Failure - Line to Neutral Voltage/1("V_LN_rms_2 ") -> [V_LN_rms_2], V_LN_rms_2/1, Divide3/1
  Power Loss/1(Ploss) -> Open Circuit/ Degradation Failure/1(Ploss)
  Failure Determination/2(DegFail) -> [DegFail]
  Failure Determination/1(OCFail) -> [OCFail]
  Fail?/1 -> Failure Determination/1(Fail?)
  Deg/1 -> Open Circuit/ Degradation Failure/4(Deg)
  [OCFail] -> Open Circuit/ Degradation Failure/3(OCFail?)
  [DegFail] -> Open Circuit/ Degradation Failure/2(DegFail?)

== system Lib_EMTAT/Components/Power Flow/AC-DC Rectifier ==
  note: V_LN_rms = V_DC
  V_LN_rms : Inport
  I_DC : Inport  Port=2
  Fail? : Inport  Port=3
  Deg : Inport  Port=4
  I_L_rms(t-1) : Inport  Port=5
  Bus Creator1 : BusCreator  Inputs=10
  Compensate for Divide By Zero. : Subsystem
  Derivative : Derivative
  Derivative1 : Derivative
  Direction Determination : Subsystem
  Divide1 : Product  Inputs=**
  Divide3 : Product  Inputs=**
  Efficiency1 : Subsystem
  Failure Determination1 : Subsystem
  Instantaneous (Total) to Average Power : Gain  Gain=1/3
  Open Circuit Failure - DC Voltage : Subsystem
  Open Circuit/ Degradation Failure : Subsystem
  Power Loss : Subsystem
  "V_DC " : Outport
  Outputs : Outport  Port=2
  Ploss : Outport  Port=3
  I_L_rms : Outport  Port=4
  I_L_rms(t) : Outport  Port=5
  wires:
  [Vdot_DC] -> Bus Creator1/6  "Vdot_DC"
  [Idot_DC] -> Bus Creator1/9  "Idot_DC"
  Derivative1/1 -> [Idot_DC]
  Derivative/1 -> [Vdot_DC]
  Open Circuit Failure - DC Voltage/1("V_DC ") -> [V_DC], Divide1/1, "V_DC "/1, Derivative/1, Divide3/1, Power Loss/1(V_DC)
  Failure Determination1/1(OCFail) -> [OCFail]
  Failure Determination1/2(DegFail) -> [DegFail]
  Fail?/1 -> Failure Determination1/1(Fail?)
  Power Loss/1(Ploss) -> Open Circuit/ Degradation Failure/1(Ploss)
  Deg/1 -> Open Circuit/ Degradation Failure/4(Deg)
  [DegFail] -> Open Circuit/ Degradation Failure/2(DegFail?)
  [OCFail] -> Open Circuit/ Degradation Failure/3(OCFail?)
  V_LN_rms/1 -> Open Circuit Failure - DC Voltage/2(V_DC), Compensate for Divide By Zero./2(V_LN_rms), [V_LN_rms]
  [OCFail] -> Open Circuit Failure - DC Voltage/1(Failed?)
  Instantaneous (Total) to Average Power/1 -> I_L_rms/1, I_L_rms(t)/1, [I_L_rms]
  I_L_rms(t-1)/1 -> Power Loss/2(I_L_rms)
  Direction Determination/1(PEquivAC) -> Compensate for Divide By Zero./1(PEquivAC)
  Bus Creator1/1 -> Outputs/1
  [P_AC] -> Bus Creator1/1  "P_AC"
  [P_DC] -> Bus Creator1/2  "P_DC"
  Open Circuit/ Degradation Failure/1("Ploss ") -> [Ploss], Direction Determination/2(Ploss)
  Divide3/1 -> [P_DC], Direction Determination/1(P_DC)
  [Ploss] -> Ploss/1
  [V_LN_rms] -> Bus Creator1/4  "V_LN_rms"
  [V_DC] -> Bus Creator1/5  "V_DC"
  [I_DC] -> Bus Creator1/8  "I_DC"
  [Ploss] -> Bus Creator1/10  "Ploss"
  [I_L_rms] -> Bus Creator1/7  "I_L_rms"
  [P_DC] -> Efficiency1/2(P_DC)
  [P_AC] -> Efficiency1/1(P_AC)
  Efficiency1/1(Eff) -> [Eff]
  [Eff] -> Bus Creator1/3  "Eff"
  Compensate for Divide By Zero./1(I_L_rms) -> Instantaneous (Total) to Average Power/1, Divide1/2
  I_DC/1 -> Divide3/2, Derivative1/1, [I_DC]
  Divide1/1 -> [P_AC]

== system Lib_EMTAT/Components/Power Flow/Cable ==
  note: Iin = Iout
  note: Memory block used to break algebraic loop.
  Vin : Inport
  Iout : Inport  Port=2
  Fail? : Inport  Port=3
  Iout(t-1) : Inport  Port=4
  Bus Creator : BusCreator  Inputs=8
  Constant : Constant  Value=R
  Divide{,1..3} (4 alike) : Product  Inputs=**
  Failure Determination : Subsystem
  Fix Zero Voltage Problem : Subsystem
  Open Circuit Failure - Current : Subsystem
  Open Circuit Failure - Voltage : Subsystem
  Square : Math  Operator=square  SaturateOnIntegerOverflow=on
  Sum : Sum  Inputs=|-+
  Vout : Outport
  Outputs : Outport  Port=2
  Ploss : Outport  Port=3
  Iin : Outport  Port=4
  Iout(t) : Outport  Port=5
  wires:
  [OCFail] -> Open Circuit Failure - Voltage/1(Failed?)
  Fix Zero Voltage Problem/1(Vout) -> Open Circuit Failure - Voltage/2(Vout)
  [OCFail] -> Open Circuit Failure - Current/1(Failed?)
  Open Circuit Failure - Current/1("Iin/Iout ") -> Iin/1, [Iin], Divide2/2, Divide3/1, Square/1
  Iout/1 -> Iout(t)/1, [Iout], Open Circuit Failure - Current/2(Iin/Iout)
  Fail?/1 -> Failure Determination/1(Fail?)
  Failure Determination/1(OCFail) -> [OCFail]
  Iout(t-1)/1 -> Divide/1
  Divide/1 -> Sum/1
  Vin/1 -> Divide2/1, Sum/2, Fix Zero Voltage Problem/2(Vin), [Vin]
  Sum/1 -> Fix Zero Voltage Problem/1("Vout "), Divide3/2
  [Iin] -> Bus Creator/3  "Iin"
  [Vout] -> Bus Creator/6  "Vout"
  [Vin] -> Bus Creator/5  "Vin"
  Bus Creator/1 -> Outputs/1
  [R] -> Bus Creator/7  "R"
  Constant/1 -> Divide1/2, [R], Divide/2
  Square/1 -> Divide1/1
  Divide1/1 -> [Ploss], Ploss/1
  [Pin] -> Bus Creator/2  "Pin"
  [Pout] -> Bus Creator/1  "Pout"
  Divide2/1 -> [Pin]
  Divide3/1 -> [Pout]
  [Ploss] -> Bus Creator/8  "Ploss"
  Open Circuit Failure - Voltage/1("Vout ") -> Vout/1, [Vout]
  [Iout] -> Bus Creator/4  "Iout"

== system Lib_EMTAT/Components/Power Flow/Current Distribution ==
  I : Inport
  Idmd : Inport  Port=2
  MATLAB Function : MATLAB Function  TreatAsAtomicUnit=on
  Isplit : Outport
  wires:
  Idmd/1 -> MATLAB Function/2(Idmd)
  MATLAB Function/1(Isplit) -> Isplit/1
  I/1 -> MATLAB Function/1(I)

== system Lib_EMTAT/Components/Power Flow/Current Junction ==
  I : Inport
  MATLAB Function : MATLAB Function  TreatAsAtomicUnit=on
  Isum : Outport
  wires:
  I/1 -> MATLAB Function/1(u)
  MATLAB Function/1(y) -> Isum/1

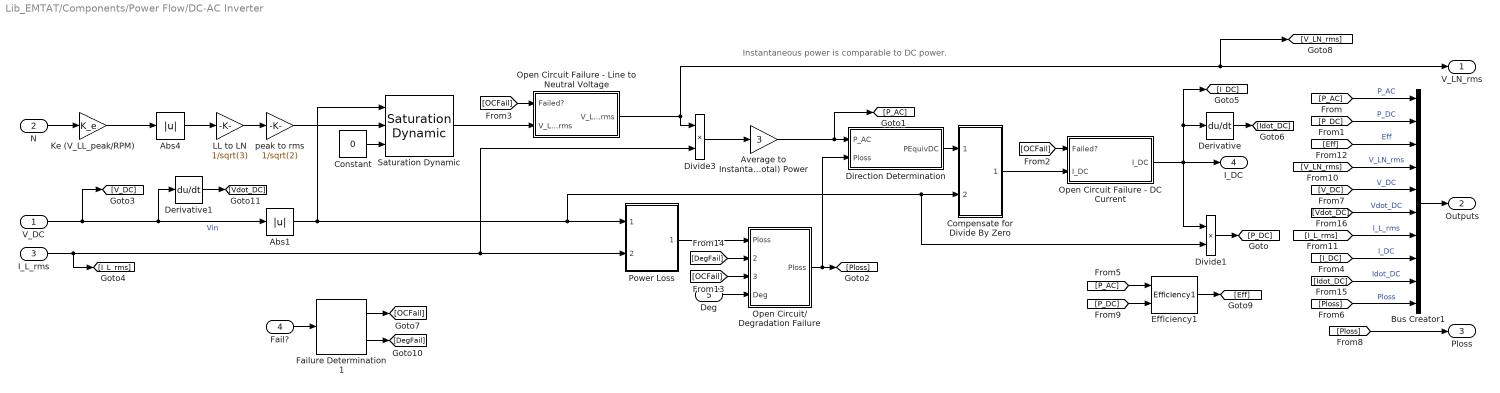
== system Lib_EMTAT/Components/Power Flow/DC-AC Inverter ==
  note: Instantaneous power is comparable to DC power.
  V_DC : Inport
  N : Inport  Port=2
  I_L_rms : Inport  Port=3
  Fail? : Inport  Port=4
  Deg : Inport  Port=5
  Abs1 : Abs
  Abs4 : Abs
  Average to Instantaneous (Total) Power : Gain  Gain=3
  Bus Creator1 : BusCreator  Inputs=10
  Compensate for Divide By Zero : Subsystem
  Constant : Constant  Value=0
  Derivative : Derivative
  Derivative1 : Derivative
  Direction Determination : Subsystem
  Divide1 : Product  Inputs=**
  Divide3 : Product  Inputs=**
  Efficiency1 : $bdroot/Components/Power Flow/AC-DC Rectifier/Efficiency1  SystemSampleTime=-1  VariantActivationTime=update diagram  Latency=0  AutoFrameSizeCalculation=off
  Failure Determination1 : $bdroot/Components/Power Flow/AC-DC Rectifier/Failure Determination1  SystemSampleTime=-1  VariantActivationTime=update diagram  Latency=0  AutoFrameSizeCalculation=off
  Ke (V_LL_peak/RPM) : Gain  Gain=K_e
  LL to LN : Gain  Gain=1/sqrt(3)
  Open Circuit Failure - DC Current : Subsystem
  Open Circuit Failure - Line to Neutral Voltage : Subsystem
  Open Circuit/ Degradation Failure : Subsystem
  Power Loss : Subsystem
  Saturation Dynamic : simulink/Discontinuities/Saturation Dynamic  OutMin=[]  OutMax=[]  OutDataTypeStr=Inherit: Same as second input  OutDataType=fixdt(1, 16)  OutScaling=2^-10  DoSatur=off
  peak to rms : Gain  Gain=1/sqrt(2)
  V_LN_rms : Outport
  Outputs : Outport  Port=2
  Ploss : Outport  Port=3
  I_DC : Outport  Port=4
  wires:
  [Vdot_DC] -> Bus Creator1/6  "Vdot_DC"
  [Idot_DC] -> Bus Creator1/9  "Idot_DC"
  Derivative1/1 -> [Vdot_DC]
  Derivative/1 -> [Idot_DC]
  [DegFail] -> Open Circuit/ Degradation Failure/2(DegFail?)
  [OCFail] -> Open Circuit/ Degradation Failure/3(OCFail?)
  Deg/1 -> Open Circuit/ Degradation Failure/4(Deg)
  Fail?/1 -> Failure Determination1/1
  Failure Determination1/1 -> [OCFail]
  Failure Determination1/2 -> [DegFail]
  Power Loss/1(Ploss) -> Open Circuit/ Degradation Failure/1(Ploss)
  Open Circuit Failure - Line to Neutral Voltage/1("V_LN_rms ") -> Divide3/1, V_LN_rms/1, [V_LN_rms]
  [OCFail] -> Open Circuit Failure - Line to Neutral Voltage/1(Failed?)
  Saturation Dynamic/1 -> Open Circuit Failure - Line to Neutral Voltage/2(V_LN_rms)
  [OCFail] -> Open Circuit Failure - DC Current/1(Failed?)
  Compensate for Divide By Zero/1(I_DC) -> Open Circuit Failure - DC Current/2(I_DC)
  LL to LN/1 -> peak to rms/1
  [Eff] -> Bus Creator1/3  "Eff"
  Efficiency1/1 -> [Eff]
  [P_AC] -> Efficiency1/1
  [P_DC] -> Efficiency1/2
  [I_L_rms] -> Bus Creator1/7  "I_L_rms"
  [Ploss] -> Bus Creator1/10  "Ploss"
  [I_DC] -> Bus Creator1/8  "I_DC"
  [V_DC] -> Bus Creator1/5  "V_DC"
  [V_LN_rms] -> Bus Creator1/4  "V_LN_rms"
  I_L_rms/1 -> [I_L_rms], Divide3/2, Power Loss/2(I_L_rms)
  [Ploss] -> Ploss/1
  Ke (V_LL_peak/RPM)/1 -> Abs4/1
  V_DC/1 -> [V_DC], Abs1/1, Derivative1/1  "Vin"
  Average to Instantaneous (Total) Power/1 -> [P_AC], Direction Determination/1(P_AC)
  Open Circuit Failure - DC Current/1("I_DC ") -> [I_DC], Derivative/1, I_DC/1, Divide1/1
  Open Circuit/ Degradation Failure/1("Ploss ") -> [Ploss], Direction Determination/2(Ploss)
  N/1 -> Ke (V_LL_peak/RPM)/1
  [P_DC] -> Bus Creator1/2  "P_DC"
  [P_AC] -> Bus Creator1/1  "P_AC"
  Bus Creator1/1 -> Outputs/1
  Direction Determination/1(PEquivDC) -> Compensate for Divide By Zero/1(PEquivDC)
  Divide1/1 -> [P_DC]
  Abs1/1 -> Saturation Dynamic/1, Divide1/2, Compensate for Divide By Zero/2(V_DC), Power Loss/1(V_DC)
  Abs4/1 -> LL to LN/1
  Divide3/1 -> Average to Instantaneous (Total) Power/1
  Constant/1 -> Saturation Dynamic/3
  peak to rms/1 -> Saturation Dynamic/2

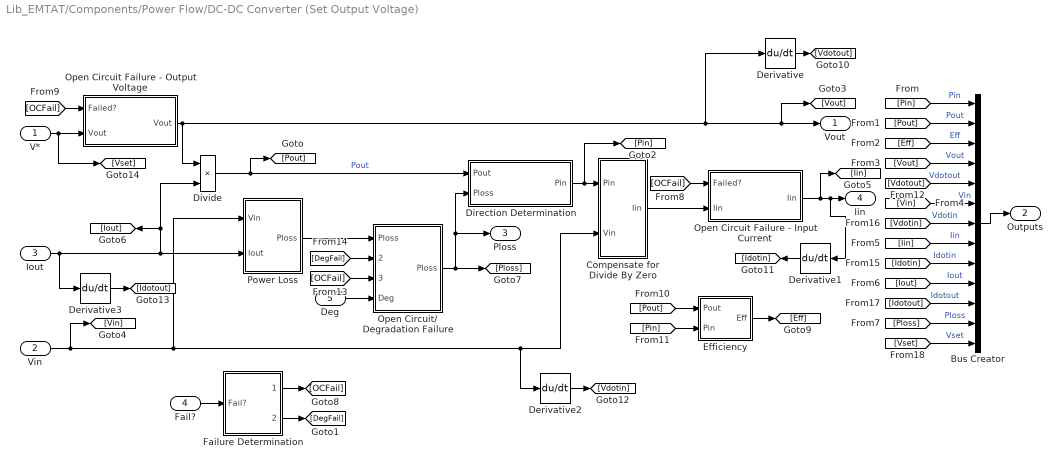
== system Lib_EMTAT/Components/Power Flow/DC-DC Converter (Set Output Voltage) ==
  V* : Inport
  Vin : Inport  Port=2
  Iout : Inport  Port=3
  Fail? : Inport  Port=4
  Deg : Inport  Port=5
  Bus Creator : BusCreator  Inputs=13
  Compensate for Divide By Zero : Subsystem
  Derivative{,1..3} (4 alike) : Derivative
  Direction Determination : Subsystem
  Divide : Product  Inputs=**
  Efficiency : Subsystem
  Failure Determination : Subsystem
  Open Circuit Failure - Input Current : Subsystem
  Open Circuit Failure - Output Voltage : Subsystem
  Open Circuit/ Degradation Failure : Subsystem
  Power Loss : Subsystem
  Vout : Outport
  Outputs : Outport  Port=2
  Ploss : Outport  Port=3
  Iin : Outport  Port=4
  wires:
  [Vset] -> Bus Creator/13  "Vset"
  [Vdotout] -> Bus Creator/5  "Vdotout"
  [Vdotin] -> Bus Creator/7  "Vdotin"
  [Idotin] -> Bus Creator/9  "Idotin"
  [Idotout] -> Bus Creator/11  "Idotout"
  Derivative3/1 -> [Idotout]
  Derivative2/1 -> [Vdotin]
  Derivative1/1 -> [Idotin]
  Derivative/1 -> [Vdotout]
  Fail?/1 -> Failure Determination/1(Fail?)
  Failure Determination/1(OCFail) -> [OCFail]
  Failure Determination/2(DegFail) -> [DegFail]
  Power Loss/1(Ploss) -> Open Circuit/ Degradation Failure/1(Ploss)
  Deg/1 -> Open Circuit/ Degradation Failure/4(Deg)
  [DegFail] -> Open Circuit/ Degradation Failure/2(DegFail?)
  [OCFail] -> Open Circuit/ Degradation Failure/3(OCFail?)
  [OCFail] -> Open Circuit Failure - Output Voltage/1(Failed?)
  Open Circuit Failure - Output Voltage/1("Vout   ") -> Divide/1, Vout/1, [Vout], Derivative/1
  [OCFail] -> Open Circuit Failure - Input Current/1(Failed?)
  Compensate for Divide By Zero/1(Iin) -> Open Circuit Failure - Input Current/2(Iin)
  Efficiency/1(Eff) -> [Eff]
  [Pin] -> Efficiency/2(Pin)
  [Pout] -> Efficiency/1(Pout)
  V*/1 -> Open Circuit Failure - Output Voltage/2(Vout), [Vset]
  Vin/1 -> [Vin], Compensate for Divide By Zero/2(Vin), Derivative2/1, Power Loss/1(Vin)
  Open Circuit Failure - Input Current/1("Iin  ") -> [Iin], Iin/1, Derivative1/1
  Open Circuit/ Degradation Failure/1("Ploss ") -> [Ploss], Direction Determination/2(Ploss), Ploss/1
  Divide/1 -> [Pout], Direction Determination/1(Pout)  "Pout"
  Bus Creator/1 -> Outputs/1
  Direction Determination/1(Pin) -> [Pin], Compensate for Divide By Zero/1(Pin)
  [Pin] -> Bus Creator/1  "Pin"
  [Pout] -> Bus Creator/2  "Pout"
  [Eff] -> Bus Creator/3  "Eff"
  [Vout] -> Bus Creator/4  "Vout"
  [Vin] -> Bus Creator/6  "Vin"
  [Iin] -> Bus Creator/8  "Iin"
  Iout/1 -> Power Loss/2(Iout), [Iout], Divide/2, Derivative3/1
  [Iout] -> Bus Creator/10  "Iout"
  [Ploss] -> Bus Creator/12  "Ploss"

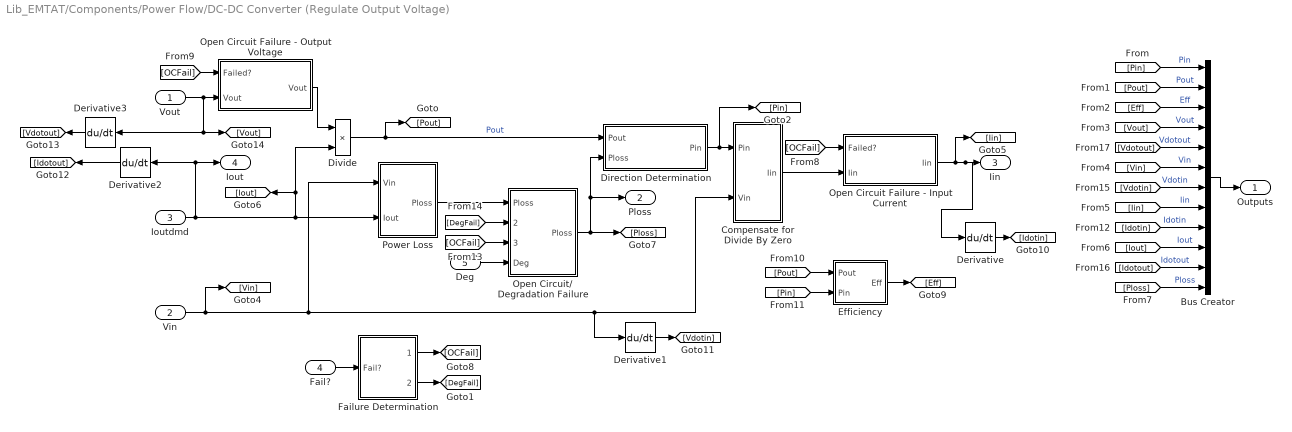
== system Lib_EMTAT/Components/Power Flow/DC-DC Converter (Regulate Output Voltage) ==
  Vout : Inport
  Vin : Inport  Port=2
  Ioutdmd : Inport  Port=3
  Fail? : Inport  Port=4
  Deg : Inport  Port=5
  Bus Creator : BusCreator  Inputs=12
  Compensate for Divide By Zero : Subsystem
  Derivative{,1..3} (4 alike) : Derivative
  Direction Determination : Subsystem
  Divide : Product  Inputs=**
  Efficiency : Subsystem
  Failure Determination : Subsystem
  Open Circuit Failure - Input Current : Subsystem
  Open Circuit Failure - Output Voltage : Subsystem
  Open Circuit/ Degradation Failure : Subsystem
  Power Loss : Subsystem
  Outputs : Outport
  Ploss : Outport  Port=2
  Iin : Outport  Port=3
  Iout : Outport  Port=4
  wires:
  [Vdotout] -> Bus Creator/5  "Vdotout"
  [Vdotin] -> Bus Creator/7  "Vdotin"
  [Idotin] -> Bus Creator/9  "Idotin"
  [Idotout] -> Bus Creator/11  "Idotout"
  Derivative3/1 -> [Vdotout]
  Derivative2/1 -> [Idotout]
  Derivative1/1 -> [Vdotin]
  Derivative/1 -> [Idotin]
  [Ploss] -> Bus Creator/12  "Ploss"
  [Iout] -> Bus Creator/10  "Iout"
  Ioutdmd/1 -> Divide/2, [Iout], Power Loss/2(Iout), Derivative2/1, Iout/1
  [Iin] -> Bus Creator/8  "Iin"
  [Vin] -> Bus Creator/6  "Vin"
  [Vout] -> Bus Creator/4  "Vout"
  [Eff] -> Bus Creator/3  "Eff"
  [Pout] -> Bus Creator/2  "Pout"
  [Pin] -> Bus Creator/1  "Pin"
  Direction Determination/1(Pin) -> Compensate for Divide By Zero/1(Pin), [Pin]
  Bus Creator/1 -> Outputs/1
  Divide/1 -> Direction Determination/1(Pout), [Pout]  "Pout"
  Open Circuit/ Degradation Failure/1("Ploss ") -> Ploss/1, Direction Determination/2(Ploss), [Ploss]
  Open Circuit Failure - Input Current/1("Iin  ") -> [Iin], Iin/1, Derivative/1
  Vin/1 -> Power Loss/1(Vin), Compensate for Divide By Zero/2(Vin), Derivative1/1, [Vin]
  Vout/1 -> Derivative3/1, [Vout], Open Circuit Failure - Output Voltage/2(Vout)
  [Pout] -> Efficiency/1(Pout)
  [Pin] -> Efficiency/2(Pin)
  Efficiency/1(Eff) -> [Eff]
  Compensate for Divide By Zero/1(Iin) -> Open Circuit Failure - Input Current/2(Iin)
  [OCFail] -> Open Circuit Failure - Input Current/1(Failed?)
  Open Circuit Failure - Output Voltage/1("Vout   ") -> Divide/1
  [OCFail] -> Open Circuit Failure - Output Voltage/1(Failed?)
  [OCFail] -> Open Circuit/ Degradation Failure/3(OCFail?)
  [DegFail] -> Open Circuit/ Degradation Failure/2(DegFail?)
  Deg/1 -> Open Circuit/ Degradation Failure/4(Deg)
  Power Loss/1(Ploss) -> Open Circuit/ Degradation Failure/1(Ploss)
  Failure Determination/2(DegFail) -> [DegFail]
  Failure Determination/1(OCFail) -> [OCFail]
  Fail?/1 -> Failure Determination/1(Fail?)

== system Lib_EMTAT/Components/Power Flow/Electrical Bus ==
  I : Inport
  V : Inport  Port=2
  "Capacitance, F" : Constant  Value=C
  Divide : Product  Inputs=*/
  MATLAB Function : MATLAB Function  TreatAsAtomicUnit=on
  "V " : Outport
  Vdot : Outport  Port=2
  wires:
  MATLAB Function/1(y) -> Divide/1
  "Capacitance, F"/1 -> Divide/2
  Divide/1 -> Vdot/1
  V/1 -> "V "/1
  I/1 -> MATLAB Function/1(u)

== system Lib_EMTAT/Components/Power Flow/Energy Storage Device ==
  note: Explanation for Convention Correction:
      | If Iout is positive, discharge the capacitor. This is because a positive current demand from a sink block means that the sink block needs current.
      | If Iout is negative, charge the capacitor. This is because a negative current demand from a sink block means that the sink block is giving current.
  "Iout " : Inport
  V : Inport  Port=2
  Iout(t-1) : Inport  Port=3
  Bus Creator : BusCreator  Inputs=8
  Constant : Constant  Value=ESR
  Convention Correction : Gain  Gain=-1
  Discrete Derivative : simulink/Discrete/Discrete Derivative  gainval=1.0  ICPrevScaledInput=0.0  OutMin=[]  OutMax=[]  OutDataType=fixdt(1, 16)  OutScaling=2^-10  DoSatur=off
  Discrete Derivative1 : simulink/Discrete/Discrete Derivative  gainval=1.0  ICPrevScaledInput=0.0  OutMin=[]  OutMax=[]  OutDataType=fixdt(1, 16)  OutScaling=2^-10  DoSatur=off
  Discrete Derivative2 : simulink/Discrete/Discrete Derivative  gainval=1.0  ICPrevScaledInput=0.0  OutMin=[]  OutMax=[]  OutDataType=fixdt(1, 16)  OutScaling=2^-10  DoSatur=off
  Divide : Product  Inputs=**
  Divide1 : Product  Inputs=**
  Gain : Gain  Gain=1/C
  SOC : Subsystem
  Saturation : Saturate  UpperLimit=inf  LowerLimit=0
  Square1 : Math  Operator=square  SaturateOnIntegerOverflow=on
  Sum : Sum  Inputs=|-+
  "Voltage, V to Energy, Wh" : Subsystem
  Warnings : Subsystem
  Vout : Outport
  Outputs : Outport  Port=2
  Ploss : Outport  Port=3
  Vdot : Outport  Port=4
  Iout(t) : Outport  Port=5
  wires:
  Saturation/1 -> "Voltage, V to Energy, Wh"/1(V), Discrete Derivative2/1, Vout/1, [Vout]
  Iout(t-1)/1 -> Discrete Derivative1/1, Convention Correction/1, Divide/1
  V/1 -> Sum/2
  Divide/1 -> Sum/1
  Constant/1 -> Divide/2, Divide1/2
  Sum/1 -> Saturation/1
  [SOC] -> Warnings/1(SOC)
  [Vdotout] -> Bus Creator/5  "Vdotout"
  [SOCdot] -> Bus Creator/7  "SOCdot"
  [Idotout] -> Bus Creator/3  "Idotout"
  Discrete Derivative/1 -> [SOCdot]
  Discrete Derivative2/1 -> [Vdotout]
  Discrete Derivative1/1 -> [Idotout]
  "Voltage, V to Energy, Wh"/1(E) -> [Energy], SOC/1(Energy (W-h))
  "Iout "/1 -> [Iout], Iout(t)/1
  SOC/1(SOC) -> [SOC], Discrete Derivative/1
  [SOC] -> Bus Creator/6  "SOC"
  Divide1/1 -> [Ploss], Ploss/1
  [Ploss] -> Bus Creator/8  "Ploss"
  Square1/1 -> Divide1/1
  Bus Creator/1 -> Outputs/1
  [Vout] -> Bus Creator/4  "Vout"
  [Iout] -> Bus Creator/2  "Iout"
  [Energy] -> Bus Creator/1  "E"
  Gain/1 -> Vdot/1  "Vdot"
  Convention Correction/1 -> Gain/1, Square1/1
